simulink model "LogicalOp_SquareWaveGeneration"  (R2016a)
settings: Solver=VariableStepAuto  StartTime=0.0  StopTime=inf  RelTol=1e-3
settings Model: Creator=DELL  LastModifiedBy=DELL

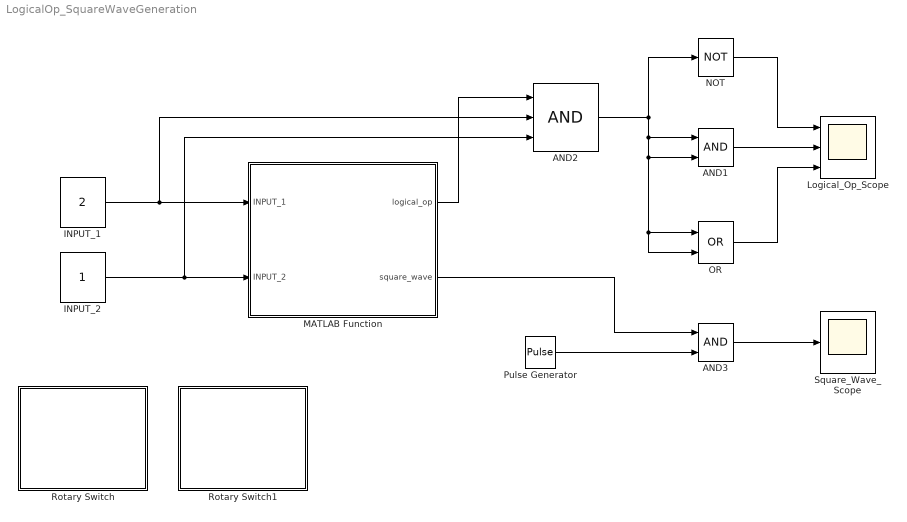
== system LogicalOp_SquareWaveGeneration ==
  AND1 : Logic  IconShape=distinctive  AllPortsSameDT=off  OutDataTypeStr=boolean
  AND2 : Logic  Inputs=3  IconShape=distinctive  AllPortsSameDT=off  OutDataTypeStr=boolean
  AND3 : Logic  IconShape=distinctive  AllPortsSameDT=off  OutDataTypeStr=boolean
  INPUT_1 : Constant  Value=2
  INPUT_2 : Constant
  Logical_Op_Scope : Scope  NumInputPorts=3
  MATLAB Function : MATLAB Function  TreatAsAtomicUnit=on
  NOT : Logic  Operator=NOT  IconShape=distinctive  AllPortsSameDT=off  OutDataTypeStr=boolean
  OR : Logic  Operator=OR  IconShape=distinctive  AllPortsSameDT=off  OutDataTypeStr=boolean
  Pulse Generator : DiscretePulseGenerator  PulseType=Time based  PulseWidth=50
  Rotary Switch : Subsystem  DialogController=hmiCreateDDGDialog  IsWebBlock=on  mask(MWDashboardBlock){webBlockId=6e8ccbfc-7208-45a1-9b4b-28e38cb516e5, webBlockType=discreteknob, ShowInLibBrowser=on, ShowInitialText=on, HMISrcModelName=LogicalOp_SquareWaveGeneration}
      mask prompts: webBlockId "WebBlock Id"; webBlockType "WebBlock Type"; HMISrcModelName "Source Model"
      mask Help: helpview([docroot '/mapfiles/simulink.map'], 'hmi_rotary_switch')
      mask Display:
      | model = bdroot(gcb);
      | if strcmp(get_param(model,'BlockDiagramType'), 'library')
      |     image([(matlabroot) '/toolbox/simulink/hmi/icons/DiscreteKnob.png']);
      | end
  Rotary Switch1 : Subsystem  DialogController=hmiCreateDDGDialog  IsWebBlock=on  mask(MWDashboardBlock){webBlockId=ce5a226f-ea24-4b71-bf36-b9cda1558e70, webBlockType=discreteknob, ShowInLibBrowser=on, ShowInitialText=on, HMISrcModelName=LogicalOp_SquareWaveGeneration}
      mask prompts: webBlockId "WebBlock Id"; webBlockType "WebBlock Type"; HMISrcModelName "Source Model"
      mask Help: helpview([docroot '/mapfiles/simulink.map'], 'hmi_rotary_switch')
      mask Display:
      | model = bdroot(gcb);
      | if strcmp(get_param(model,'BlockDiagramType'), 'library')
      |     image([(matlabroot) '/toolbox/simulink/hmi/icons/DiscreteKnob.png']);
      | end
  Square_Wave_Scope : Scope
  wires:
  INPUT_1/1 -> AND2/2, MATLAB Function/1(INPUT_1)
  INPUT_2/1 -> AND2/3, MATLAB Function/2(INPUT_2)
  MATLAB Function/1(logical_op) -> AND2/1
  AND2/1 -> AND1/1, AND1/2, OR/1, OR/2, NOT/1
  NOT/1 -> Logical_Op_Scope/1
  AND1/1 -> Logical_Op_Scope/2
  OR/1 -> Logical_Op_Scope/3
  MATLAB Function/2(square_wave) -> AND3/1
  Pulse Generator/1 -> AND3/2
  AND3/1 -> Square_Wave_Scope/1

== system LogicalOp_SquareWaveGeneration/Rotary Switch ==

== system LogicalOp_SquareWaveGeneration/Rotary Switch1 ==

== matlab function LogicalOp_SquareWaveGeneration/MATLAB Function ==
  data: INPUT_1 input; logical_op output; INPUT_2 input; square_wave output
function [logical_op,square_wave] = My_Func(INPUT_1,INPUT_2)
%#codegen
  if INPUT_1 == 1 && INPUT_2 == 1
     logical_op = 1;
     square_wave = 0;
  else 
     logical_op = 0;
     square_wave = 1;
     while 1 
        if INPUT_1 ~= 1 || INPUT_2 ~= 1
            break
        end    
     end   
  end   
end
